simulink model "VU_lineFollow2"  (Simulink 7.5)
settings: Solver=FixedStepDiscrete  StartTime=0.0  StopTime=inf  FixedStep=0.1  RelTol=1e-3
libraries: lego_nxt_lib x4
settings Model: Creator=jpeytonj  LastModifiedBy=jpeytonj
settings RTWCC: SystemTargetFile=lrt.tlc  GenCodeOnly=on  TemplateMakefile=lrt_ecrobot.tmf  Description=Lego NXT Real-Time Target  ProcessScript=lrt_make_rtw_hook
settings STFCustomTargetCC: ModelReferenceCompliant=off  GeneratePreprocessorConditionals=Disable all  MatFileLogging=on  SystemTargetFile=lrt.tlc
settings GRTTargetCC: ModelReferenceCompliant=off  ParMdlRefBuildCompliant=off  CompOptLevelCompliant=off  ExtModeMexFile=noextcomm
settings CustomProperty: DataType=RTWOptions_EnumType_C__RTtools_VU-LRT_lrt_1codeGenType  Value=Integer-only
settings EnumStrPairs: String=Integer-only

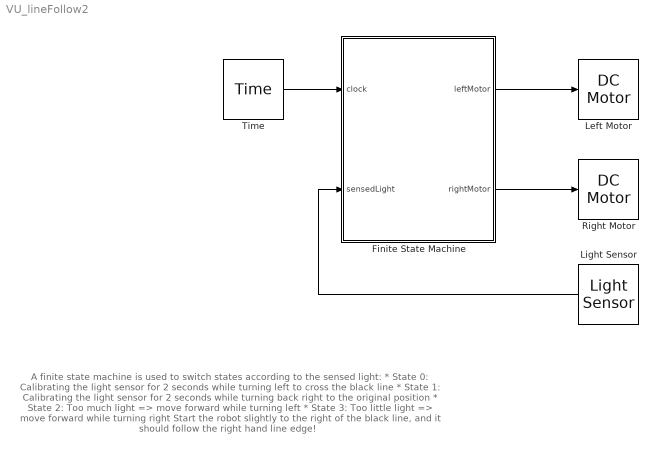
== system VU_lineFollow2 ==
  note: A finite state machine is used to switch states according to the sensed light:
      | * State 0:  Calibrating the light sensor for 2 seconds while turning left to cross the black line
      | * State 1:  Calibrating the light sensor for 2 seconds while turning back right to the original position
      | * State 2:  Too much light => move forward while turning left
      | * State 3:  Too little light => move forward while turning right
      | Start the robot slightly to the right of the black line, and it should follow the right hand line edge!
  Finite State Machine : Stateflow chart  TreatAsAtomicUnit=on
  Left Motor : lego_nxt_lib/DC Motor  port=Port C  brake=Coast
  Light Sensor : lego_nxt_lib/Light Sensor  port=Port 3  st=0.1
  Right Motor : lego_nxt_lib/DC Motor  port=Port B  brake=Coast
  Time : lego_nxt_lib/Time  st=0.1
  wires:
  Time/1 -> Finite State Machine/1(clock)
  Finite State Machine/1(leftMotor) -> Left Motor/1
  Finite State Machine/2(rightMotor) -> Right Motor/1
  Light Sensor/1 -> Finite State Machine/2(sensedLight)

== stateflow chart Finite State Machine ==
  state S0_Calib1
    entry:
    leftMotor= int8(-60);
    rightMotor= int8(60);
    during:
    if (sensedLight<minLight),
    minLight=sensedLight;
    end;
    if (sensedLight>maxLight),
    maxLight=sensedLight;
    end;
  state S1_Calib2
    entry:
    leftMotor= int8(-60);
    rightMotor= int8(60);
    during:
    if sensedLight<minLight,
    minLight=sensedLight;
    end;
    if sensedLight>maxLight,
    maxLight=sensedLight;
    end;
    exit:
    threshold = (minLight+maxLight) /2;
  state S2_TooBright
    entry:
    leftMotor= int8(55);
    rightMotor= int8(65);
  state S3_TooDark
    entry:
    leftMotor= int8(65);
    rightMotor= int8(55);
  S0_Calib1 -> S1_Calib2 : [clock>2000]
  S1_Calib2 -> S2_TooBright : [clock>4000]
  S2_TooBright -> S3_TooDark : [sensedLight>threshold]
  S3_TooDark -> S2_TooBright : [sensedLight<threshold]
  (default) -> S0_Calib1
  data: clock input double; sensedLight input double; leftMotor output int8; rightMotor output int8; threshold local uint16 size=1 =45; minLight local uint16 size=1 =1023; maxLight local uint16 size=1 =0
